simulink model "PubIfDecisionLM_MDL"  (R2020b)
settings: configuration reference "DspaceConfig" (kept outside this file)
PostLoadFcn:
  | if any(exist('dsrtsu_mdlpostloadfcn', 'file') ~= 0), dsrtsu_mdlpostloadfcn('Execute', bdroot); end
InitFcn:
  | , if any(exist('dsmpb_private', 'file') ~= 0), dsmpb_private('dsmpb_mdlclblib', 'Init', bdroot); end,
undefined symbols (not defined in the file or in its folder): OFM_OBJ_FUSIONTYPE_E, OFM_OBJ_MOVINGSTATE_E, OFM_OBJ_ORIENTATION_E, OFM_OBJ_TYPE_E, P_LM_Cyc, P_LM_EMLHistKapRcdBufSize, P_LM_EMLHistTrajBaseDis, P_LM_EMLHistTrajPNum, P_LM_EMLKapCorrMaxThre, P_LM_EMLMinKapThre, P_LM_EMLPathDisDiffThre, P_LM_EMLQuaFiltPar, P_LM_EMLTurnActKapThre, P_LM_EMLValidQuaThre, P_LM_FntPath1Disgap, P_LM_FntPath1MinDis, P_LM_FntPath1Timegap, P_LM_FntPath2Disgap, P_LM_FntPath2MinDis, P_LM_FntPath2Timegap, P_LM_FntPath3Disgap, P_LM_FntPath3MinDis, P_LM_FntPath3Timegap, P_LM_FusBLParFiltP, P_LM_FusEVDifC2Thre, P_LM_FusEVOPath1AllVSLDisThre, P_LM_FusEVOPath1AllVSLLostNumThre, P_LM_FusEVOPath1AllVSLQuaThre, P_LM_FusEVOPath1OTLFacNLC, P_LM_FusOTLQuaThre, P_LM_FusOTLSW, P_LM_FusParC0Index, P_LM_FusParC1Index, P_LM_FusParC2Index, P_LM_FusParC3Index, P_LM_FusVSLQuaThre, P_LM_FusVSLSW, P_LM_FusVSLValidSteerWheerAngThre, P_LM_FusVSLValidVxvThre, P_LM_LaneWidth, P_LM_OTLBufTPInfoEvaFactor, P_LM_OTLObjNum, P_LM_OTLObjSelectAgeThre, P_LM_OTLObjSelectDxAssessVx, P_LM_OTLObjSelectDxThre, P_LM_OTLObjSelectVxThre, P_LM_OTLObjSelectVyAssessDx, P_LM_OTLObjSelectVyThre, P_LM_OTLTrajPntBaseDis, P_LM_OTLTrajStdThre, P_LM_VSLAvailLineNum, P_LM_VSLBLSDiffThre, P_LM_VSLBLSDisRatio, P_LM_VSLFusBLParFiltP_C1, P_LM_VSLFusBLParFiltP_C2, P_LM_VSLFusBLParFiltP_C3, P_LM_VSLFusBLParFiltP_Quality, P_LM_VSLHistTrajBaseDis, P_LM_VSLHistTrajPNum, P_LM_VSLLCC0diff ... (+18)
libraries: simulink x145, LM_LIB x43
(part 13 of 24)

== system PubIfDecisionLM_MDL/Subsystem2/LM_OTL/LM_OTL_MovObjTrajRecord3/LM_OTL_MovObjSelc/LM_OTL_MovObjInterestedSelc/LM_OTL_ObjSelcIndexCalc ==
  ObjSelcDxInfo : Inport
  ObjSelcDyInfo : Inport  Port=2
  C_LM_ObjNum : Inport  Port=3
  LM_OTL_ObjSelcCalc : Subsystem
  LM_OTL_ObjSelcInfoOpt : Subsystem
  LeObj1CheckInfo : Outport
  LeObj2CheckInfo : Outport  Port=2
  HostObj1CheckInfo : Outport  Port=3
  HostObj2CheckInfo : Outport  Port=4
  RigObj1CheckInfo : Outport  Port=5
  RigObj2CheckInfo : Outport  Port=6
  wires:
  LM_OTL_ObjSelcCalc/4(HostObj2CheckInfo) -> HostObj2CheckInfo/1
  LM_OTL_ObjSelcCalc/1(LeObj1CheckInfo) -> LeObj1CheckInfo/1
  C_LM_ObjNum/1 -> LM_OTL_ObjSelcCalc/4(C_LM_ObjNum)
  ObjSelcDxInfo/1 -> LM_OTL_ObjSelcInfoOpt/1(ObjSelcDxInfo)
  LM_OTL_ObjSelcCalc/2(LeObj2CheckInfo) -> LeObj2CheckInfo/1
  ObjSelcDyInfo/1 -> LM_OTL_ObjSelcInfoOpt/2(ObjSelcDyInfo)
  LM_OTL_ObjSelcInfoOpt/3(RigObjSlecDxInfo) -> LM_OTL_ObjSelcCalc/3(RigObjSlecDxInfo)
  LM_OTL_ObjSelcInfoOpt/1(LeObjSelcDxInfo) -> LM_OTL_ObjSelcCalc/1(LeObjSelcDxInfo)
  LM_OTL_ObjSelcCalc/6(RigObj2CheckInfo) -> RigObj2CheckInfo/1
  LM_OTL_ObjSelcInfoOpt/2(HostObjSlecDxInfo) -> LM_OTL_ObjSelcCalc/2(HostObjSlecDxInfo)
  LM_OTL_ObjSelcCalc/5(RigObj1CheckInfo) -> RigObj1CheckInfo/1
  LM_OTL_ObjSelcCalc/3(HostObj1CheckInfo) -> HostObj1CheckInfo/1

== system PubIfDecisionLM_MDL/Subsystem2/LM_OTL/LM_OTL_MovObjTrajRecord3/LM_OTL_MovObjSelc/LM_OTL_MovObjInterestedSelc/LM_OTL_ObjSelcIndexCheck ==
  LeObj1CheckInfo : Inport
  LeObj2CheckInfo : Inport  Port=2
  HostObj1CheckInfo : Inport  Port=3
  HostObj2CheckInfo : Inport  Port=4
  RigObj1CheckInfo : Inport  Port=5
  RigObj2CheckInfo : Inport  Port=6
  LM_OTL_MovObjValid : Inport  Port=7
  Object_DX : Inport  Port=8
  HostObj1Check : Subsystem
  HostObj2Check : Subsystem
  LeObj1Check : Subsystem
  LeObj2Check : Subsystem
  RigObj1Check : Subsystem
  RigObj2Check : Subsystem
  LM_OTLLeObj1Index : Outport  PortDimensions=1
  LM_OTLLeObj2Index : Outport  Port=2  PortDimensions=1
  LM_OTLHostObj1Index : Outport  Port=3  PortDimensions=1
  LM_OTLHostObj2Index : Outport  Port=4  PortDimensions=1
  LM_OTLRigObj1Index : Outport  Port=5  PortDimensions=1
  LM_OTLRigObj2Index : Outport  Port=6  PortDimensions=1
  wires:
  LM_OTL_MovObjValid/1 -> RigObj2Check/1(LM_OTL_MovObjValid), RigObj1Check/1(LM_OTL_MovObjValid), HostObj2Check/1(LM_OTL_MovObjValid), HostObj1Check/1(LM_OTL_MovObjValid), LeObj2Check/1(LM_OTL_MovObjValid), LeObj1Check/1(LM_OTL_MovObjValid)
  Object_DX/1 -> LeObj1Check/2(Object_DX), LeObj2Check/2(Object_DX), HostObj1Check/2(Object_DX), HostObj2Check/2(Object_DX), RigObj1Check/2(Object_DX), RigObj2Check/2(Object_DX)
  RigObj2CheckInfo/1 -> RigObj2Check/3(RigObj2CheckInfo)
  RigObj2Check/1(LM_OTLRigObj2Index) -> LM_OTLRigObj2Index/1
  RigObj1CheckInfo/1 -> RigObj1Check/3(RigObj1CheckInfo)
  RigObj1Check/1(LM_OTLRigObj1Index) -> LM_OTLRigObj1Index/1
  HostObj2CheckInfo/1 -> HostObj2Check/3(HostObj2CheckInfo)
  HostObj2Check/1(LM_OTLHostObj2Index) -> LM_OTLHostObj2Index/1
  HostObj1CheckInfo/1 -> HostObj1Check/3(HostObj1CheckInfo)
  HostObj1Check/1(LM_OTLHostObj1Index) -> LM_OTLHostObj1Index/1
  LeObj2CheckInfo/1 -> LeObj2Check/3(LeObj2CheckInfo)
  LeObj2Check/1(LM_OTLLeObj2Index) -> LM_OTLLeObj2Index/1
  LeObj1Check/1(LM_OTLLeObj1Index) -> LM_OTLLeObj1Index/1
  LeObj1CheckInfo/1 -> LeObj1Check/3(LeObj1CheckInfo)

== system PubIfDecisionLM_MDL/Subsystem2/LM_OTL/LM_OTL_MovObjTrajRecord3/LM_OTL_MovObjSelc/LM_OTL_MovObjInterestedSelc/LM_OTL_ObjSelcInfoCalc ==
  ILM_OTL_MovObjValid : Inport
  Object_DX : Inport  Port=2
  Object_DY : Inport  Port=3
  C_LM_ObjNum : Inport  Port=4
  Constant1 : Constant  Value=255  OutDataTypeStr=single
  Constant2 : Constant  Value=255  OutDataTypeStr=single
  Index Vector : MultiPortSwitch  Inputs=1
  Index Vector1 : MultiPortSwitch  Inputs=1
  Index Vector2 : MultiPortSwitch  Inputs=1
  Switch6 : Switch  Criteria=u2 > Threshold
  Switch7 : Switch  Criteria=u2 > Threshold
  ObjSelcDxInfo : Outport
  ObjSelcDyInfo : Outport  Port=2
  wires:
  ILM_OTL_MovObjValid/1 -> Index Vector/2
  Object_DY/1 -> Index Vector2/2
  Switch6/1 -> ObjSelcDxInfo/1
  Constant2/1 -> Switch7/3
  Index Vector/1 -> Switch6/2, Switch7/2
  C_LM_ObjNum/1 -> Index Vector/1, Index Vector1/1, Index Vector2/1
  Index Vector1/1 -> Switch6/1
  Object_DX/1 -> Index Vector1/2
  Constant1/1 -> Switch6/3
  Switch7/1 -> ObjSelcDyInfo/1
  Index Vector2/1 -> Switch7/1

== system PubIfDecisionLM_MDL/Subsystem2/LM_OTL/LM_OTL_MovObjTrajRecord3/LM_OTL_MovObjSelc/Subsystem3/ILM_OTL_MovObjSelectDeFault ==
  Action Port : ActionPort  ActionPortLabel=if(u1)
  Constant : Constant  Value=0  OutDataTypeStr=boolean
  LM_OTL_MovObjValid : Outport
  wires:
  Constant/1 -> LM_OTL_MovObjValid/1

== system PubIfDecisionLM_MDL/Subsystem2/LM_OTL/LM_OTL_MovObjTrajRecord3/LM_OTL_MovObjSelc/Subsystem3/LM_OTL_MovObjSelect ==
  vxvRefMs : Inport
  Object_Type : Inport  Port=2
  Object_MovingState : Inport  Port=3
  Object_VX : Inport  Port=4
  Object_Orientation : Inport  Port=5
  Object_Fus_Type : Inport  Port=6
  Object_ExistProb : Inport  Port=7
  Object_VY : Inport  Port=8
  Object_DX : Inport  Port=9
  Object_Age : Inport  Port=10
  Action Port : ActionPort  ActionPortLabel=else
  LM_OTL_ExistProbAssess : Subsystem
  LM_OTL_FusTypeAssess : Subsystem
  LM_OTL_MovDirAssess : Subsystem
  LM_OTL_MovStsAssess : Subsystem
  LM_OTL_ObjAgeAssess : Subsystem
  LM_OTL_ObjDxAssess : Subsystem
  LM_OTL_ObjTypeAssess : Subsystem
  LM_OTL_ObjVyAssess : Subsystem
  Logical Operator : Logic  Inputs=8  AllPortsSameDT=off  OutDataTypeStr=boolean
  LM_OTL_MovObjValid : Outport
  wires:
  LM_OTL_ObjTypeAssess/1(LM_OTL_ObjTypeAssess) -> Logical Operator/1
  Object_Type/1 -> LM_OTL_ObjTypeAssess/1(Object_Type)
  LM_OTL_ObjDxAssess/1(LM_OTL_ObjDxValid) -> Logical Operator/7
  LM_OTL_ObjAgeAssess/1(LM_OTL_ObjAgeValid) -> Logical Operator/8
  LM_OTL_ObjVyAssess/1(LM_OTL_ObjVyValid) -> Logical Operator/6
  LM_OTL_ExistProbAssess/1(LM_OTL_ExistProbValid) -> Logical Operator/5
  LM_OTL_FusTypeAssess/1(LM_OTL_FusTypeValid) -> Logical Operator/4
  LM_OTL_MovDirAssess/1(LM_OTL_MovDirValid) -> Logical Operator/3
  LM_OTL_MovStsAssess/1(LM_OTL_MovStsValid) -> Logical Operator/2
  Object_VX/1 -> LM_OTL_MovStsAssess/2(Object_VX)
  Object_DX/1 -> LM_OTL_ObjVyAssess/2(Object_DX), LM_OTL_ObjDxAssess/1(Object_DX)
  Object_Orientation/1 -> LM_OTL_MovDirAssess/1(Object_Orientation)
  Object_MovingState/1 -> LM_OTL_MovStsAssess/1(Object_MovingState)
  Object_Age/1 -> LM_OTL_ObjAgeAssess/1(Object_Age)
  Object_Fus_Type/1 -> LM_OTL_FusTypeAssess/1(Object_Fus_Type), LM_OTL_ExistProbAssess/1(Object_Fus_Type)
  Logical Operator/1 -> LM_OTL_MovObjValid/1
  Object_ExistProb/1 -> LM_OTL_ExistProbAssess/2(Object_ExistProb)
  Object_VY/1 -> LM_OTL_ObjVyAssess/1(Object_VY)
  vxvRefMs/1 -> LM_OTL_MovStsAssess/3(vxvRefMs), LM_OTL_ObjDxAssess/2(vxvRefMs)

== system PubIfDecisionLM_MDL/Subsystem2/LM_OTL/LM_OTL_MovObjTrajRecord3/LM_OTL_MovObjSelc/Subsystem3/ObjIsInvalidCalc ==
  ObjectID : Inport
  Compare To Constant : simulink/Logic and Bit Operations/Compare To Constant  relop===  const=0  OutDataTypeStr=boolean
  ObjIsInvalid : Outport
  wires:
  Compare To Constant/1 -> ObjIsInvalid/1
  ObjectID/1 -> Compare To Constant/1

== system PubIfDecisionLM_MDL/Subsystem2/LM_OTL/LM_OTL_MovObjTrajRecord3/LM_OTL_ObjAlreadyRcdedJudge/LM_OTL_CurObjIDCalc/LM_OTL_CurEgoLaObjID ==
  Object_ID : Inport  BusOutputAsStruct=on
  LM_OTLCurEgoLaObj1Index : Inport  Port=2
  LM_OTLCurEgoLaObj2Index : Inport  Port=3
  Compare To Zero : simulink/Logic and Bit Operations/Compare To Zero  relop===  OutDataTypeStr=boolean
  Compare To Zero1 : simulink/Logic and Bit Operations/Compare To Zero  relop===  OutDataTypeStr=boolean
  Constant : Constant  Value=0  OutDataTypeStr=uint8
  Constant1 : Constant  OutDataTypeStr=uint8
  Constant2 : Constant  Value=0  OutDataTypeStr=uint8
  Constant3 : Constant  OutDataTypeStr=uint8
  Index Vector2 : MultiPortSwitch  Inputs=1
  Index Vector3 : MultiPortSwitch  Inputs=1
  Switch{,1..3} (4 alike) : Switch  Criteria=u2 ~= 0
  LM_OTLCurEgoLaObj1ID : Outport
  LM_OTLCurEgoLaObj2ID : Outport  Port=2
  wires:
  Switch1/1 -> Index Vector2/1
  LM_OTLCurEgoLaObj1Index/1 -> Switch1/3, Compare To Zero/1
  Constant/1 -> Switch/1
  Index Vector3/1 -> Switch2/3  "LM_Ego2ObjID"
  Compare To Zero1/1 -> Switch2/2, Switch3/2
  Constant3/1 -> Switch3/1
  Index Vector2/1 -> Switch/3  "LM_Ego1ObjID"
  Object_ID/1 -> Index Vector3/2, Index Vector2/2
  Switch/1 -> LM_OTLCurEgoLaObj1ID/1  "LM_OTLCurEgoLaObj1ID"
  LM_OTLCurEgoLaObj2Index/1 -> Compare To Zero1/1, Switch3/3
  Switch2/1 -> LM_OTLCurEgoLaObj2ID/1  "LM_OTLCurEgoLaObj2ID"
  Compare To Zero/1 -> Switch1/2, Switch/2
  Constant2/1 -> Switch2/1
  Switch3/1 -> Index Vector3/1
  Constant1/1 -> Switch1/1

== system PubIfDecisionLM_MDL/Subsystem2/LM_OTL/LM_OTL_MovObjTrajRecord3/LM_OTL_ObjAlreadyRcdedJudge/LM_OTL_CurObjIDCalc/LM_OTL_CurLeLaObjID ==
  Object_ID : Inport  BusOutputAsStruct=on
  LM_OTLCurLeLaObj1Index : Inport  Port=2
  LM_OTLCurLeLaObj2Index : Inport  Port=3
  Compare To Zero : simulink/Logic and Bit Operations/Compare To Zero  relop===  OutDataTypeStr=boolean
  Compare To Zero1 : simulink/Logic and Bit Operations/Compare To Zero  relop===  OutDataTypeStr=boolean
  Constant : Constant  Value=0  OutDataTypeStr=uint8
  Constant1 : Constant  OutDataTypeStr=uint8
  Constant2 : Constant  Value=0  OutDataTypeStr=uint8
  Constant3 : Constant  OutDataTypeStr=uint8
  Index Vector2 : MultiPortSwitch  Inputs=1
  Index Vector3 : MultiPortSwitch  Inputs=1
  Switch{,1..3} (4 alike) : Switch  Criteria=u2 ~= 0
  LM_OTLCurLeLaObj1ID : Outport
  LM_OTLCurLeLaObj2ID : Outport  Port=2
  wires:
  Index Vector3/1 -> Switch2/3  "LM_Le2ObjID"
  Index Vector2/1 -> Switch/3  "LM_Le1ObjID"
  Object_ID/1 -> Index Vector3/2, Index Vector2/2
  LM_OTLCurLeLaObj1Index/1 -> Switch1/3, Compare To Zero/1
  Compare To Zero/1 -> Switch1/2, Switch/2
  Switch/1 -> LM_OTLCurLeLaObj1ID/1  "LM_OTLCurLeLaObj1ID"
  Constant/1 -> Switch/1
  Switch1/1 -> Index Vector2/1
  Constant1/1 -> Switch1/1
  Constant2/1 -> Switch2/1
  Switch2/1 -> LM_OTLCurLeLaObj2ID/1  "LM_OTLCurLeLaObj2ID"
  Constant3/1 -> Switch3/1
  Compare To Zero1/1 -> Switch2/2, Switch3/2
  LM_OTLCurLeLaObj2Index/1 -> Compare To Zero1/1, Switch3/3
  Switch3/1 -> Index Vector3/1

== system PubIfDecisionLM_MDL/Subsystem2/LM_OTL/LM_OTL_MovObjTrajRecord3/LM_OTL_ObjAlreadyRcdedJudge/LM_OTL_CurObjIDCalc/LM_OTL_RigEgoLaObjID ==
  Object_ID : Inport  BusOutputAsStruct=on
  LM_OTLCurRigLaObj1Index : Inport  Port=2
  LM_OTLCurRigLaObj2Index : Inport  Port=3
  Compare To Zero : simulink/Logic and Bit Operations/Compare To Zero  relop===  OutDataTypeStr=boolean
  Compare To Zero1 : simulink/Logic and Bit Operations/Compare To Zero  relop===  OutDataTypeStr=boolean
  Constant : Constant  Value=0  OutDataTypeStr=uint8
  Constant1 : Constant  OutDataTypeStr=uint8
  Constant2 : Constant  Value=0  OutDataTypeStr=uint8
  Constant3 : Constant  OutDataTypeStr=uint8
  Index Vector2 : MultiPortSwitch  Inputs=1
  Index Vector3 : MultiPortSwitch  Inputs=1
  Switch{,1..3} (4 alike) : Switch  Criteria=u2 ~= 0
  LM_OTLCurRigLaObj1ID : Outport
  LM_OTLCurRigLaObj2ID : Outport  Port=2
  wires:
  Constant/1 -> Switch/1
  Compare To Zero1/1 -> Switch2/2, Switch3/2
  Index Vector3/1 -> Switch2/3  "LM_Rig2ObjID"
  Switch1/1 -> Index Vector2/1
  LM_OTLCurRigLaObj1Index/1 -> Switch1/3, Compare To Zero/1
  Constant1/1 -> Switch1/1
  Compare To Zero/1 -> Switch1/2, Switch/2
  Switch3/1 -> Index Vector3/1
  Constant2/1 -> Switch2/1
  Object_ID/1 -> Index Vector3/2, Index Vector2/2
  Switch/1 -> LM_OTLCurRigLaObj1ID/1  "LM_OTLCurRigLaObj1ID"
  Constant3/1 -> Switch3/1
  Index Vector2/1 -> Switch/3  "LM_Rig1ObjID"
  LM_OTLCurRigLaObj2Index/1 -> Compare To Zero1/1, Switch3/3
  Switch2/1 -> LM_OTLCurRigLaObj2ID/1  "LM_OTLCurRigLaObj2ID"

== system PubIfDecisionLM_MDL/Subsystem2/LM_OTL/LM_OTL_MovObjTrajRecord3/LM_OTL_ObjRcdFlgJudge/LM_OTL_CurObjDxCalc/LM_OTLCurEgoLaObjDxCalc ==
  LM_OTLCurEgoLaObj1Index : Inport
  Object_Dx : Inport  Port=2
  Object_Dy : Inport  Port=3
  LM_OTLCurEgoLaObj2Index : Inport  Port=4
  Compare To Zero : simulink/Logic and Bit Operations/Compare To Zero  relop===  OutDataTypeStr=boolean
  Compare To Zero1 : simulink/Logic and Bit Operations/Compare To Zero  relop===  OutDataTypeStr=boolean
  Constant : Constant  Value=0  OutDataTypeStr=single
  Constant8 : Constant  OutDataTypeStr=uint8
  Constant9 : Constant  OutDataTypeStr=uint8
  Index Vector{1..4} (4 alike) : MultiPortSwitch  Inputs=1
  Switch{1..6} (6 alike) : Switch  Criteria=u2 ~= 0
  LM_OTLCurEgoLaObj1Dx : Outport
  LM_OTLCurEgoLaObj1Dy : Outport  Port=2
  LM_OTLCurEgoLaObj2Dx : Outport  Port=3
  LM_OTLCurEgoLaObj2Dy : Outport  Port=4
  wires:
  Index Vector4/1 -> Switch4/3
  Switch4/1 -> LM_OTLCurEgoLaObj2Dy/1  "LM_OTLCurEgoLaObj2Dy"
  Index Vector1/1 -> Switch3/3
  Object_Dy/1 -> Index Vector1/2, Index Vector4/2
  Switch3/1 -> LM_OTLCurEgoLaObj1Dy/1  "LM_OTLCurEgoLaObj1Dy"
  Index Vector3/1 -> Switch2/3
  Constant/1 -> Switch1/1, Switch2/1, Switch4/1, Switch3/1
  Switch1/1 -> LM_OTLCurEgoLaObj1Dx/1  "LM_OTLCurEgoLaObj1Dx"
  Switch2/1 -> LM_OTLCurEgoLaObj2Dx/1  "LM_OTLCurEgoLaObj2Dx"
  Index Vector2/1 -> Switch1/3
  Switch5/1 -> Index Vector2/1, Index Vector1/1
  Switch6/1 -> Index Vector3/1, Index Vector4/1
  Constant9/1 -> Switch6/1
  Compare To Zero/1 -> Switch5/2, Switch1/2, Switch3/2
  Compare To Zero1/1 -> Switch6/2, Switch2/2, Switch4/2
  Constant8/1 -> Switch5/1
  Object_Dx/1 -> Index Vector3/2, Index Vector2/2
  LM_OTLCurEgoLaObj1Index/1 -> Compare To Zero/1, Switch5/3
  LM_OTLCurEgoLaObj2Index/1 -> Switch6/3, Compare To Zero1/1

== system PubIfDecisionLM_MDL/Subsystem2/LM_OTL/LM_OTL_MovObjTrajRecord3/LM_OTL_ObjRcdFlgJudge/LM_OTL_CurObjDxCalc/LM_OTLCurLeLaObjDxCalc ==
  LM_OTLCurLeLaObj1Index : Inport
  Object_Dx : Inport  Port=2
  Object_Dy : Inport  Port=3
  LM_OTLCurLeLaObj2Index : Inport  Port=4
  Compare To Zero : simulink/Logic and Bit Operations/Compare To Zero  relop===  OutDataTypeStr=boolean
  Compare To Zero1 : simulink/Logic and Bit Operations/Compare To Zero  relop===  OutDataTypeStr=boolean
  Constant : Constant  Value=0  OutDataTypeStr=single
  Constant8 : Constant  OutDataTypeStr=uint8
  Constant9 : Constant  OutDataTypeStr=uint8
  Index Vector{1..4} (4 alike) : MultiPortSwitch  Inputs=1
  Switch{1..6} (6 alike) : Switch  Criteria=u2 ~= 0
  LM_OTLCurLeLaObj1Dx : Outport
  LM_OTLCurLeLaObj1Dy : Outport  Port=2
  LM_OTLCurLeLaObj2Dx : Outport  Port=3
  LM_OTLCurLeLaObj2Dy : Outport  Port=4
  wires:
  LM_OTLCurLeLaObj2Index/1 -> Compare To Zero1/1, Switch6/3
  LM_OTLCurLeLaObj1Index/1 -> Switch5/3, Compare To Zero/1
  Object_Dx/1 -> Index Vector2/2, Index Vector3/2
  Constant8/1 -> Switch5/1
  Compare To Zero1/1 -> Switch4/2, Switch2/2, Switch6/2
  Compare To Zero/1 -> Switch3/2, Switch1/2, Switch5/2
  Constant9/1 -> Switch6/1
  Switch6/1 -> Index Vector4/1, Index Vector3/1
  Switch5/1 -> Index Vector1/1, Index Vector2/1
  Index Vector2/1 -> Switch1/3
  Switch2/1 -> LM_OTLCurLeLaObj2Dx/1  "LM_OTLCurLeLaObj2Dx"
  Switch1/1 -> LM_OTLCurLeLaObj1Dx/1  "LM_OTLCurLeLaObj1Dx"
  Constant/1 -> Switch3/1, Switch4/1, Switch2/1, Switch1/1
  Index Vector3/1 -> Switch2/3
  Switch3/1 -> LM_OTLCurLeLaObj1Dy/1  "LM_OTLCurLeLaObj1Dy"
  Object_Dy/1 -> Index Vector4/2, Index Vector1/2
  Index Vector1/1 -> Switch3/3
  Switch4/1 -> LM_OTLCurLeLaObj2Dy/1  "LM_OTLCurLeLaObj2Dy"
  Index Vector4/1 -> Switch4/3

== system PubIfDecisionLM_MDL/Subsystem2/LM_OTL/LM_OTL_MovObjTrajRecord3/LM_OTL_ObjRcdFlgJudge/LM_OTL_CurObjDxCalc/LM_OTLCurRigLaObjDxCalc ==
  LM_OTLCurRigLaObj1Index : Inport
  Object_Dx : Inport  Port=2
  Object_Dy : Inport  Port=3
  LM_OTLCurRigLaObj2Index : Inport  Port=4
  Compare To Zero : simulink/Logic and Bit Operations/Compare To Zero  relop===  OutDataTypeStr=boolean
  Compare To Zero1 : simulink/Logic and Bit Operations/Compare To Zero  relop===  OutDataTypeStr=boolean
  Constant : Constant  Value=0  OutDataTypeStr=single
  Constant8 : Constant  OutDataTypeStr=uint8
  Constant9 : Constant  OutDataTypeStr=uint8
  Index Vector{1..4} (4 alike) : MultiPortSwitch  Inputs=1
  Switch{1..6} (6 alike) : Switch  Criteria=u2 ~= 0
  LM_OTLCurRigLaObj1Dx : Outport
  LM_OTLCurRigLaObj1Dy : Outport  Port=2
  LM_OTLCurRigLaObj2Dx : Outport  Port=3
  LM_OTLCurRigLaObj2Dy : Outport  Port=4
  wires:
  LM_OTLCurRigLaObj2Index/1 -> Compare To Zero1/1, Switch6/3
  LM_OTLCurRigLaObj1Index/1 -> Switch5/3, Compare To Zero/1
  Object_Dx/1 -> Index Vector2/2, Index Vector3/2
  Constant8/1 -> Switch5/1
  Compare To Zero1/1 -> Switch4/2, Switch2/2, Switch6/2
  Compare To Zero/1 -> Switch3/2, Switch1/2, Switch5/2
  Constant9/1 -> Switch6/1
  Switch6/1 -> Index Vector4/1, Index Vector3/1
  Switch5/1 -> Index Vector1/1, Index Vector2/1
  Index Vector2/1 -> Switch1/3
  Switch2/1 -> LM_OTLCurRigLaObj2Dx/1  "LM_OTLCurRigLaObj2Dx"
  Switch1/1 -> LM_OTLCurRigLaObj1Dx/1  "LM_OTLCurRigLaObj1Dx"
  Constant/1 -> Switch3/1, Switch4/1, Switch2/1, Switch1/1
  Index Vector3/1 -> Switch2/3
  Switch3/1 -> LM_OTLCurRigLaObj1Dy/1  "LM_OTLCurRigLaObj1Dy"
  Object_Dy/1 -> Index Vector4/2, Index Vector1/2
  Index Vector1/1 -> Switch3/3
  Switch4/1 -> LM_OTLCurRigLaObj2Dy/1  "LM_OTLCurRigLaObj2Dy"
  Index Vector4/1 -> Switch4/3

== system PubIfDecisionLM_MDL/Subsystem2/LM_OTL/LM_OTL_MovObjTrajRecord3/LM_OTL_ObjStoreInfoCalc/LM_OTL_BufLe1InfoUpdate1/LM_OTL_BufLe1InfoUpdate ==
  LM_OTLBufL1DxVectK1Adju : Inport
  LM_OTLBufL1DyVectK1Adju : Inport  Port=2
  LM_OTLBufL1UpdateFlg : Inport  Port=3
  LM_OTLBufL1Objdx : Inport  Port=4
  LM_OTLBufL1Objdy : Inport  Port=5
  LM_OTLBufL1EPPos : Inport  Port=6
  If : If  IfExpression=u1 ~= 0
  If Action Subsystem : Subsystem  TreatAsAtomicUnit=on
  If Action Subsystem1 : Subsystem  TreatAsAtomicUnit=on
  Merge : Merge
  Merge1 : Merge
  LM_OTLBufL1DxVect : Outport  PortDimensions=80
  LM_OTLBufL1DyVect : Outport  Port=2  PortDimensions=80
  wires:
  Merge1/1 -> LM_OTLBufL1DyVect/1  "LM_OTLBufL1DyVect"
  If Action Subsystem1/2(LM_OTLBufL1DyVect) -> Merge1/2
  If Action Subsystem/2(LM_OTLBufL1DyVect) -> Merge1/1
  Merge/1 -> LM_OTLBufL1DxVect/1  "LM_OTLBufL1DxVect"
  If Action Subsystem1/1(LM_OTLBufL1DxVect) -> Merge/2
  If Action Subsystem/1(LM_OTLBufL1DxVect) -> Merge/1
  LM_OTLBufL1EPPos/1 -> If Action Subsystem/3(LM_OTLBufL1EPPos)
  LM_OTLBufL1Objdy/1 -> If Action Subsystem/2(LM_OTLBufL1Objdy)
  LM_OTLBufL1Objdx/1 -> If Action Subsystem/1(LM_OTLBufL1Objdx)
  LM_OTLBufL1DyVectK1Adju/1 -> If Action Subsystem1/2(LM_OTLBufL1DyVectK1Adju), If Action Subsystem/5(LM_OTLBufL1DyVectK1Adju)
  LM_OTLBufL1DxVectK1Adju/1 -> If Action Subsystem1/1(LM_OTLBufL1DxVectK1Adju), If Action Subsystem/4(LM_OTLBufL1DxVectK1Adju)
  If/2 -> If Action Subsystem1/Action
  If/1 -> If Action Subsystem/Action
  LM_OTLBufL1UpdateFlg/1 -> If/1

== system PubIfDecisionLM_MDL/Subsystem2/LM_OTL/LM_OTL_MovObjTrajRecord3/LM_OTL_ObjStoreInfoCalc/LM_OTL_BufLe1InfoUpdate1/LM_OTL_BufLe1StoreInfoCalc ==
  LM_OTLBufIndex : Inport
  LM_OTLCurLeLaObj1RcdedFlg : Inport  Port=2
  LM_OTLCurLeLaObj2RcdedFlg : Inport  Port=3
  LM_OTLCurLeLaObj1RcdFlg : Inport  Port=4
  LM_OTLCurLeLaObj2RcdFlg : Inport  Port=5
  LM_OTLCurLeLaObj1ID : Inport  Port=6
  LM_OTLCurLeLaObj2ID : Inport  Port=7
  LM_OTLCurLeLaObj1Dx : Inport  Port=8
  LM_OTLCurLeLaObj2Dx : Inport  Port=9
  LM_OTLCurLeLaObj1Dy : Inport  Port=10
  LM_OTLCurLeLaObj2Dy : Inport  Port=11
  LM_OTLBufL1PNumK1 : Inport  Port=12
  LM_OTLBufL1SPPosK1 : Inport  Port=13
  LM_OTLBufL1EPPosK1 : Inport  Port=14
  LM_OTLCurLeLaObj1Index : Inport  Port=15
  LM_OTLCurLeLaObj2Index : Inport  Port=16
  LM_OTLBufL1LastTPValid : Inport  Port=17
  LM_OTLBufL1LastEPPos : Inport  Port=18
  If : If  NumInputs=3  IfExpression=u1 == u2  ElseIfExpressions=u2 == u3
  LM_OTL_ObjSICCurLeObj1InBufLe1 : Subsystem
  LM_OTL_ObjSICCurLeObj2InBufLe1 : Subsystem
  LM_OTL_ObjSICNoCurObjInBufLe1 : Subsystem
  Merge{,1..6} (7 alike) : Merge  Inputs=3
  LM_OTLBufL1UpdateFlg : Outport
  LM_OTLBufL1Objdx : Outport  Port=2
  LM_OTLBufL1Objdy : Outport  Port=3
  LM_OTLBufL1EPPos : Outport  Port=4
  LM_OTLBufL1ObjID : Outport  Port=5
  LM_OTLBufL1ObjTPNum : Outport  Port=6
  LM_OTLBufL1SPPos : Outport  Port=7
  wires:
  LM_OTLBufIndex/1 -> If/1
  If/1 -> LM_OTL_ObjSICCurLeObj1InBufLe1/Action
  If/2 -> LM_OTL_ObjSICCurLeObj2InBufLe1/Action
  If/3 -> LM_OTL_ObjSICNoCurObjInBufLe1/Action
  LM_OTLCurLeLaObj1RcdedFlg/1 -> LM_OTL_ObjSICNoCurObjInBufLe1/3(LM_OTLCurLeLaObj1RcdedFlg), If/2
  LM_OTLCurLeLaObj2RcdedFlg/1 -> If/3
  LM_OTLCurLeLaObj1RcdFlg/1 -> LM_OTL_ObjSICCurLeObj1InBufLe1/1(LM_OTLCurLeLaObj1RcdFlg)
  LM_OTLCurLeLaObj1ID/1 -> LM_OTL_ObjSICNoCurObjInBufLe1/4(LM_OTLCurLeLaObj1ID), LM_OTL_ObjSICCurLeObj1InBufLe1/2(LM_OTLCurLeLaObj1ID)
  LM_OTLCurLeLaObj1Dx/1 -> LM_OTL_ObjSICNoCurObjInBufLe1/6(LM_OTLCurLeLaObj1Dx), LM_OTL_ObjSICCurLeObj1InBufLe1/3(LM_OTLCurLeLaObj1Dx)
  LM_OTLCurLeLaObj1Dy/1 -> LM_OTL_ObjSICNoCurObjInBufLe1/8(LM_OTLCurLeLaObj1Dy), LM_OTL_ObjSICCurLeObj1InBufLe1/4(LM_OTLCurLeLaObj1Dy)
  LM_OTLBufL1PNumK1/1 -> LM_OTL_ObjSICCurLeObj2InBufLe1/5(LM_OTLBufL1PNumK1), LM_OTL_ObjSICCurLeObj1InBufLe1/5(LM_OTLBufL1PNumK1)
  LM_OTLBufL1SPPosK1/1 -> LM_OTL_ObjSICCurLeObj2InBufLe1/6(LM_OTLBufL1SPPosK1), LM_OTL_ObjSICCurLeObj1InBufLe1/6(LM_OTLBufL1SPPosK1)
  LM_OTLBufL1EPPosK1/1 -> LM_OTL_ObjSICCurLeObj2InBufLe1/7(LM_OTLBufL1EPPosK1), LM_OTL_ObjSICCurLeObj1InBufLe1/7(LM_OTLBufL1EPPosK1)
  LM_OTLCurLeLaObj2RcdFlg/1 -> LM_OTL_ObjSICCurLeObj2InBufLe1/1(LM_OTLCurLeLaObj2RcdFlg)
  LM_OTLCurLeLaObj2ID/1 -> LM_OTL_ObjSICCurLeObj2InBufLe1/2(LM_OTLCurLeLaObj2ID), LM_OTL_ObjSICNoCurObjInBufLe1/5(LM_OTLCurLeLaObj2ID)
  LM_OTLCurLeLaObj2Dx/1 -> LM_OTL_ObjSICNoCurObjInBufLe1/7(LM_OTLCurLeLaObj2Dx), LM_OTL_ObjSICCurLeObj2InBufLe1/3(LM_OTLCurLeLaObj2Dx)
  LM_OTLCurLeLaObj2Dy/1 -> LM_OTL_ObjSICNoCurObjInBufLe1/9(LM_OTLCurLeLaObj2Dy), LM_OTL_ObjSICCurLeObj2InBufLe1/4(LM_OTLCurLeLaObj2Dy)
  LM_OTL_ObjSICCurLeObj1InBufLe1/1(LM_OTLBufL1UpdateFlg) -> Merge/1
  Merge/1 -> LM_OTLBufL1UpdateFlg/1
  LM_OTL_ObjSICCurLeObj1InBufLe1/2(LM_OTLBufL1ObjID) -> Merge1/1
  Merge1/1 -> LM_OTLBufL1ObjID/1
  LM_OTL_ObjSICCurLeObj1InBufLe1/3(LM_OTLBufL1Objdx) -> Merge2/1
  Merge2/1 -> LM_OTLBufL1Objdx/1
  LM_OTL_ObjSICCurLeObj1InBufLe1/4(LM_OTLBufL1Objdy) -> Merge3/1
  Merge3/1 -> LM_OTLBufL1Objdy/1
  LM_OTL_ObjSICCurLeObj1InBufLe1/5(LM_OTLBufL1ObjTPNum) -> Merge4/1
  Merge4/1 -> LM_OTLBufL1ObjTPNum/1
  LM_OTL_ObjSICCurLeObj1InBufLe1/6(LM_OTLBufL1ObjTPSP) -> Merge5/1
  Merge5/1 -> LM_OTLBufL1SPPos/1
  LM_OTL_ObjSICCurLeObj1InBufLe1/7(LM_OTLBufL1ObjTPEP) -> Merge6/1
  Merge6/1 -> LM_OTLBufL1EPPos/1
  LM_OTL_ObjSICCurLeObj2InBufLe1/1(LM_OTLBufL1UpdateFlg) -> Merge/2
  LM_OTL_ObjSICCurLeObj2InBufLe1/2(LM_OTLBufL1ObjID) -> Merge1/2
  LM_OTL_ObjSICCurLeObj2InBufLe1/3(LM_OTLBufL1Objdx) -> Merge2/2
  LM_OTL_ObjSICCurLeObj2InBufLe1/4(LM_OTLBufL1Objdy) -> Merge3/2
  LM_OTL_ObjSICCurLeObj2InBufLe1/5(LM_OTLBufL1ObjTPNum) -> Merge4/2
  LM_OTL_ObjSICCurLeObj2InBufLe1/6(LM_OTLBufL1ObjTPSP) -> Merge5/2
  LM_OTL_ObjSICCurLeObj2InBufLe1/7(LM_OTLBufL1ObjTPEP) -> Merge6/2
  LM_OTL_ObjSICNoCurObjInBufLe1/1(LM_OTLBufL1UpdateFlg) -> Merge/3
  LM_OTL_ObjSICNoCurObjInBufLe1/2(LM_OTLBufL1ObjID) -> Merge1/3
  LM_OTL_ObjSICNoCurObjInBufLe1/3(LM_OTLBufL1Objdx) -> Merge2/3
  LM_OTL_ObjSICNoCurObjInBufLe1/4(LM_OTLBufL1Objdy) -> Merge3/3
  LM_OTL_ObjSICNoCurObjInBufLe1/5(LM_OTLBufL1ObjTPNum) -> Merge4/3
  LM_OTL_ObjSICNoCurObjInBufLe1/6(LM_OTLBufL1ObjTPSP) -> Merge5/3
  LM_OTL_ObjSICNoCurObjInBufLe1/7(LM_OTLBufL1ObjTPEP) -> Merge6/3
  LM_OTLCurLeLaObj1Index/1 -> LM_OTL_ObjSICNoCurObjInBufLe1/1(LM_OTLCurLeLaObj1Index)
  LM_OTLCurLeLaObj2Index/1 -> LM_OTL_ObjSICNoCurObjInBufLe1/2(LM_OTLCurLeLaObj2Index)
  LM_OTLBufL1LastTPValid/1 -> LM_OTL_ObjSICNoCurObjInBufLe1/10(LM_OTLBufL1LastTPValid)
  LM_OTLBufL1LastEPPos/1 -> LM_OTL_ObjSICNoCurObjInBufLe1/11(LM_OTLBufL1LastEPPos)

== system PubIfDecisionLM_MDL/Subsystem2/LM_OTL/LM_OTL_MovObjTrajRecord3/LM_OTL_ObjStoreInfoCalc/Subsystem/LM_OTL_BufEPPosInfo ==
  LM_OTLBufL1EPPos : Inport
  LM_OTLBufL2EPPos : Inport  Port=2
  LM_OTLBufE1EPPos : Inport  Port=3
  LM_OTLBufE2EPPos : Inport  Port=4
  LM_OTLBufR1EPPos : Inport  Port=5
  LM_OTLBufR2EPPos : Inport  Port=6
  Bus Creator5 : BusCreator  Inputs=6
  LM_OTLBufEPPosInfo : Outport
  wires:
  Bus Creator5/1 -> LM_OTLBufEPPosInfo/1  "LM_OTLBufEPPosInfo"
  LM_OTLBufL2EPPos/1 -> Bus Creator5/2  "LM_OTLBufL2EPPos"
  LM_OTLBufR2EPPos/1 -> Bus Creator5/6  "LM_OTLBufR2EPPos"
  LM_OTLBufR1EPPos/1 -> Bus Creator5/5  "LM_OTLBufR1EPPos"
  LM_OTLBufL1EPPos/1 -> Bus Creator5/1  "LM_OTLBufL1EPPos"
  LM_OTLBufE2EPPos/1 -> Bus Creator5/4  "LM_OTLBufE2EPPos"
  LM_OTLBufE1EPPos/1 -> Bus Creator5/3  "LM_OTLBufE1EPPos"

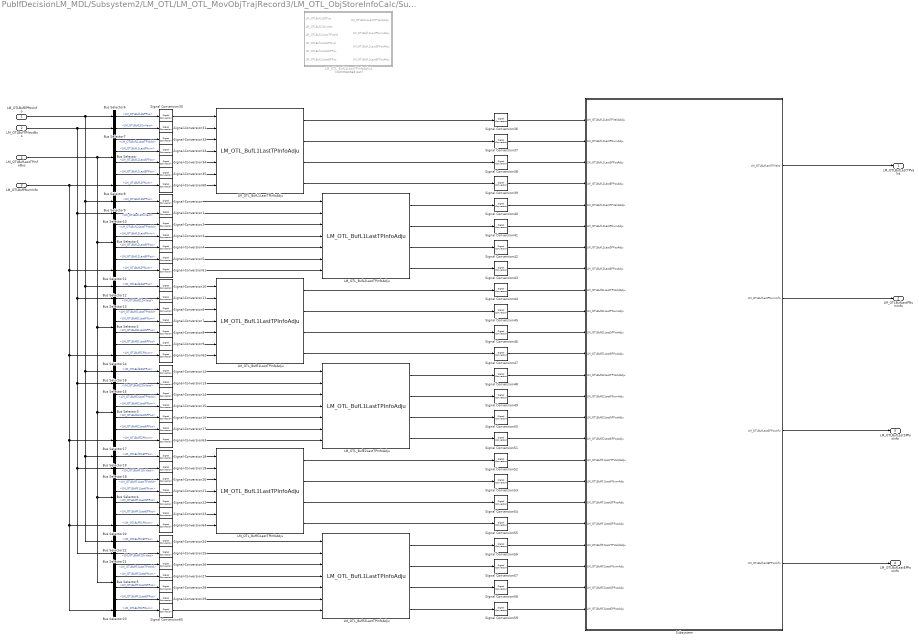
== system PubIfDecisionLM_MDL/Subsystem2/LM_OTL/LM_OTL_MovObjTrajRecord3/LM_OTL_ObjStoreInfoCalc/Subsystem/LM_OTL_BufLastTPInfo ==
  LM_OTLBufEPPosInfo : Inport
  LM_OTLBufTPVectBus : Inport  Port=2
  LM_OTLBufPNumInfo : Inport  Port=3
  LM_OTLBufLastTPInfoBus : Inport  Port=4
  Bus Selector : BusSelector  OutputSignals=LM_OTLBufL1LastTPInfo.LM_OTLBufL1LastTPValid,LM_OTLBufL1LastTPInfo.LM_OTLBufL1LastPNum,LM_OTLBufL1LastTPInfo.LM_OTLBufL1LastSPPos,LM_OTLBufL1LastTPInfo.LM_OTLBufL1LastEPPos
  Bus Selector1 : BusSelector  OutputSignals=LM_OTLBufL2LastTPInfo.LM_OTLBufL2LastTPValid,LM_OTLBufL2LastTPInfo.LM_OTLBufL2LastPNum,LM_OTLBufL2LastTPInfo.LM_OTLBufL2LastSPPos,LM_OTLBufL2LastTPInfo.LM_OTLBufL2LastEPPos
  Bus Selector10 : BusSelector  OutputSignals=LM_OTLBufL2DxVect
  Bus Selector11 : BusSelector  OutputSignals=LM_OTLBufL2PNum
  Bus Selector12 : BusSelector  OutputSignals=LM_OTLBufE1EPPos
  Bus Selector13 : BusSelector  OutputSignals=LM_OTLBufE1DxVect
  Bus Selector14 : BusSelector  OutputSignals=LM_OTLBufE1PNum
  Bus Selector15 : BusSelector  OutputSignals=LM_OTLBufE2DxVect
  Bus Selector16 : BusSelector  OutputSignals=LM_OTLBufE2EPPos
  Bus Selector17 : BusSelector  OutputSignals=LM_OTLBufE2PNum
  Bus Selector18 : BusSelector  OutputSignals=LM_OTLBufR1DxVect
  Bus Selector19 : BusSelector  OutputSignals=LM_OTLBufR1EPPos
  Bus Selector2 : BusSelector  OutputSignals=LM_OTLBufE1LastTPInfo.LM_OTLBufE1LastTPValid,LM_OTLBufE1LastTPInfo.LM_OTLBufE1LastPNum,LM_OTLBufE1LastTPInfo.LM_OTLBufE1LastSPPos,LM_OTLBufE1LastTPInfo.LM_OTLBufE1LastEPPos
  Bus Selector20 : BusSelector  OutputSignals=LM_OTLBufR1PNum
  Bus Selector21 : BusSelector  OutputSignals=LM_OTLBufR2DxVect
  Bus Selector22 : BusSelector  OutputSignals=LM_OTLBufR2EPPos
  Bus Selector23 : BusSelector  OutputSignals=LM_OTLBufR2PNum
  Bus Selector3 : BusSelector  OutputSignals=LM_OTLBufE2LastTPInfo.LM_OTLBufE2LastTPValid,LM_OTLBufE2LastTPInfo.LM_OTLBufE2LastPNum,LM_OTLBufE2LastTPInfo.LM_OTLBufE2LastSPPos,LM_OTLBufE2LastTPInfo.LM_OTLBufE2LastEPPos
  Bus Selector4 : BusSelector  OutputSignals=LM_OTLBufR1LastTPInfo.LM_OTLBufR1LastTPValid,LM_OTLBufR1LastTPInfo.LM_OTLBufR1LastPNum,LM_OTLBufR1LastTPInfo.LM_OTLBufR1LastSPPos,LM_OTLBufR1LastTPInfo.LM_OTLBufR1LastEPPos
  Bus Selector5 : BusSelector  OutputSignals=LM_OTLBufR2LastTPInfo.LM_OTLBufR2LastTPValid,LM_OTLBufR2LastTPInfo.LM_OTLBufR2LastPNum,LM_OTLBufR2LastTPInfo.LM_OTLBufR2LastSPPos,LM_OTLBufR2LastTPInfo.LM_OTLBufR2LastEPPos
  Bus Selector6 : BusSelector  OutputSignals=LM_OTLBufL1EPPos
  Bus Selector7 : BusSelector  OutputSignals=LM_OTLBufL1DxVect
  Bus Selector8 : BusSelector  OutputSignals=LM_OTLBufL1PNum
  Bus Selector9 : BusSelector  OutputSignals=LM_OTLBufL2EPPos
  LM_OTL_BufE1LastTPInfoAdju : LM_LIB/LM_OTL_BufL1LastTPInfoAdju  SystemSampleTime=-1  VariantActivationTime=update diagram  Latency=0  AutoFrameSizeCalculation=off
  LM_OTL_BufE2LastTPInfoAdju : LM_LIB/LM_OTL_BufL1LastTPInfoAdju  SystemSampleTime=-1  VariantActivationTime=update diagram  Latency=0  AutoFrameSizeCalculation=off
  LM_OTL_BufL1LastTPInfoAdju : LM_LIB/LM_OTL_BufL1LastTPInfoAdju  SystemSampleTime=-1  VariantActivationTime=update diagram  Latency=0  AutoFrameSizeCalculation=off
  LM_OTL_BufL1LastTPInfoAdju1 : Subsystem  Commented=on
  LM_OTL_BufL2LastTPInfoAdju : LM_LIB/LM_OTL_BufL1LastTPInfoAdju  SystemSampleTime=-1  VariantActivationTime=update diagram  Latency=0  AutoFrameSizeCalculation=off
  LM_OTL_BufR1LastTPInfoAdju : LM_LIB/LM_OTL_BufL1LastTPInfoAdju  SystemSampleTime=-1  VariantActivationTime=update diagram  Latency=0  AutoFrameSizeCalculation=off
  LM_OTL_BufR2LastTPInfoAdju : LM_LIB/LM_OTL_BufL1LastTPInfoAdju  SystemSampleTime=-1  VariantActivationTime=update diagram  Latency=0  AutoFrameSizeCalculation=off
  Signal Conversion{,1..65} (66 alike) : SignalConversion  OverrideOpt=off
  Subsystem : Subsystem
  LM_OTLBufLastTPValid : Outport
  LM_OTLBufLastPNumInfo : Outport  Port=2
  LM_OTLBufLastSPPosInfo : Outport  Port=3
  LM_OTLBufLastEPPosInfo : Outport  Port=4
  wires:
  Signal Conversion65/1 -> LM_OTL_BufR2LastTPInfoAdju/7
  Bus Selector23/1 -> Signal Conversion65/1  "<LM_OTLBufR2PNum>"
  Bus Selector21/1 -> Signal Conversion25/1  "<LM_OTLBufR2DxVect>"
  Bus Selector22/1 -> Signal Conversion24/1  "<LM_OTLBufR2EPPos>"
  LM_OTLBufTPVectBus/1 -> Bus Selector7/1, Bus Selector10/1, Bus Selector13/1, Bus Selector15/1, Bus Selector18/1, Bus Selector21/1
  LM_OTLBufEPPosInfo/1 -> Bus Selector6/1, Bus Selector9/1, Bus Selector12/1, Bus Selector16/1, Bus Selector19/1, Bus Selector22/1
  Signal Conversion64/1 -> LM_OTL_BufR1LastTPInfoAdju/7
  Bus Selector20/1 -> Signal Conversion64/1  "<LM_OTLBufR1PNum>"
  Bus Selector19/1 -> Signal Conversion18/1  "<LM_OTLBufR1EPPos>"
  Bus Selector18/1 -> Signal Conversion19/1  "<LM_OTLBufR1DxVect>"
  Signal Conversion63/1 -> LM_OTL_BufE2LastTPInfoAdju/7
  Bus Selector17/1 -> Signal Conversion63/1  "<LM_OTLBufE2PNum>"
  Bus Selector15/1 -> Signal Conversion13/1  "<LM_OTLBufE2DxVect>"
  Bus Selector16/1 -> Signal Conversion12/1  "<LM_OTLBufE2EPPos>"
  Signal Conversion62/1 -> LM_OTL_BufE1LastTPInfoAdju/7
  Bus Selector14/1 -> Signal Conversion62/1  "<LM_OTLBufE1PNum>"
  Signal Conversion61/1 -> LM_OTL_BufL2LastTPInfoAdju/7
  Bus Selector11/1 -> Signal Conversion61/1  "<LM_OTLBufL2PNum>"
  Bus Selector10/1 -> Signal Conversion1/1  "<LM_OTLBufL2DxVect>"
  Bus Selector9/1 -> Signal Conversion/1  "<LM_OTLBufL2EPPos>"
  LM_OTLBufPNumInfo/1 -> Bus Selector8/1, Bus Selector11/1, Bus Selector14/1, Bus Selector17/1, Bus Selector23/1, Bus Selector20/1
  Bus Selector8/1 -> Signal Conversion60/1  "<LM_OTLBufL1PNum>"
  Bus Selector7/1 -> Signal Conversion31/1  "<LM_OTLBufL1DxVect>"
  Bus Selector6/1 -> Signal Conversion30/1  "<LM_OTLBufL1EPPos>"
  Signal Conversion60/1 -> LM_OTL_BufL1LastTPInfoAdju/7
  Bus Selector/1 -> Signal Conversion32/1  "<LM_OTLBufL1LastTPValid>"
  Bus Selector/2 -> Signal Conversion33/1  "<LM_OTLBufL1LastPNum>"
  Bus Selector/3 -> Signal Conversion34/1  "<LM_OTLBufL1LastSPPos>"
  Bus Selector/4 -> Signal Conversion35/1  "<LM_OTLBufL1LastEPPos>"
  Signal Conversion/1 -> LM_OTL_BufL2LastTPInfoAdju/1
  Signal Conversion1/1 -> LM_OTL_BufL2LastTPInfoAdju/2
  Bus Selector1/2 -> Signal Conversion3/1  "<LM_OTLBufL2LastPNum>"
  Bus Selector1/1 -> Signal Conversion2/1  "<LM_OTLBufL2LastTPValid>"
  Bus Selector1/3 -> Signal Conversion4/1  "<LM_OTLBufL2LastSPPos>"
  Bus Selector1/4 -> Signal Conversion5/1  "<LM_OTLBufL2LastEPPos>"
  Bus Selector12/1 -> Signal Conversion10/1  "<LM_OTLBufE1EPPos>"
  Bus Selector13/1 -> Signal Conversion11/1  "<LM_OTLBufE1DxVect>"
  Signal Conversion2/1 -> LM_OTL_BufL2LastTPInfoAdju/3
  Signal Conversion3/1 -> LM_OTL_BufL2LastTPInfoAdju/4
  Signal Conversion4/1 -> LM_OTL_BufL2LastTPInfoAdju/5
  Signal Conversion5/1 -> LM_OTL_BufL2LastTPInfoAdju/6
  Signal Conversion9/1 -> LM_OTL_BufE1LastTPInfoAdju/6
  Signal Conversion8/1 -> LM_OTL_BufE1LastTPInfoAdju/5
  Signal Conversion7/1 -> LM_OTL_BufE1LastTPInfoAdju/4
  Signal Conversion6/1 -> LM_OTL_BufE1LastTPInfoAdju/3
  Bus Selector2/4 -> Signal Conversion9/1  "<LM_OTLBufE1LastEPPos>"
  Bus Selector2/3 -> Signal Conversion8/1  "<LM_OTLBufE1LastSPPos>"
  Bus Selector2/1 -> Signal Conversion6/1  "<LM_OTLBufE1LastTPValid>"
  Bus Selector2/2 -> Signal Conversion7/1  "<LM_OTLBufE1LastPNum>"
  Signal Conversion10/1 -> LM_OTL_BufE1LastTPInfoAdju/1
  Signal Conversion11/1 -> LM_OTL_BufE1LastTPInfoAdju/2
  Signal Conversion13/1 -> LM_OTL_BufE2LastTPInfoAdju/2
  Signal Conversion12/1 -> LM_OTL_BufE2LastTPInfoAdju/1
  Bus Selector3/2 -> Signal Conversion15/1  "<LM_OTLBufE2LastPNum>"
  Bus Selector3/1 -> Signal Conversion14/1  "<LM_OTLBufE2LastTPValid>"
  Bus Selector3/3 -> Signal Conversion16/1  "<LM_OTLBufE2LastSPPos>"
  Bus Selector3/4 -> Signal Conversion17/1  "<LM_OTLBufE2LastEPPos>"
  Signal Conversion14/1 -> LM_OTL_BufE2LastTPInfoAdju/3
  Signal Conversion15/1 -> LM_OTL_BufE2LastTPInfoAdju/4
  Signal Conversion16/1 -> LM_OTL_BufE2LastTPInfoAdju/5
  Signal Conversion17/1 -> LM_OTL_BufE2LastTPInfoAdju/6
  Signal Conversion23/1 -> LM_OTL_BufR1LastTPInfoAdju/6
  Signal Conversion22/1 -> LM_OTL_BufR1LastTPInfoAdju/5
  Signal Conversion21/1 -> LM_OTL_BufR1LastTPInfoAdju/4
  Signal Conversion20/1 -> LM_OTL_BufR1LastTPInfoAdju/3
  Bus Selector4/4 -> Signal Conversion23/1  "<LM_OTLBufR1LastEPPos>"
  Bus Selector4/3 -> Signal Conversion22/1  "<LM_OTLBufR1LastSPPos>"
  Bus Selector4/1 -> Signal Conversion20/1  "<LM_OTLBufR1LastTPValid>"
  Bus Selector4/2 -> Signal Conversion21/1  "<LM_OTLBufR1LastPNum>"
  Signal Conversion18/1 -> LM_OTL_BufR1LastTPInfoAdju/1
  Signal Conversion19/1 -> LM_OTL_BufR1LastTPInfoAdju/2
  Signal Conversion25/1 -> LM_OTL_BufR2LastTPInfoAdju/2
  Signal Conversion24/1 -> LM_OTL_BufR2LastTPInfoAdju/1
  LM_OTLBufLastTPInfoBus/1 -> Bus Selector/1, Bus Selector1/1, Bus Selector2/1, Bus Selector3/1, Bus Selector4/1, Bus Selector5/1
  Bus Selector5/2 -> Signal Conversion27/1  "<LM_OTLBufR2LastPNum>"
  Bus Selector5/1 -> Signal Conversion26/1  "<LM_OTLBufR2LastTPValid>"
  Bus Selector5/3 -> Signal Conversion28/1  "<LM_OTLBufR2LastSPPos>"
  Bus Selector5/4 -> Signal Conversion29/1  "<LM_OTLBufR2LastEPPos>"
  Signal Conversion26/1 -> LM_OTL_BufR2LastTPInfoAdju/3
  Signal Conversion27/1 -> LM_OTL_BufR2LastTPInfoAdju/4
  Signal Conversion28/1 -> LM_OTL_BufR2LastTPInfoAdju/5
  Signal Conversion29/1 -> LM_OTL_BufR2LastTPInfoAdju/6
  Signal Conversion30/1 -> LM_OTL_BufL1LastTPInfoAdju/1
  Signal Conversion31/1 -> LM_OTL_BufL1LastTPInfoAdju/2
  Signal Conversion32/1 -> LM_OTL_BufL1LastTPInfoAdju/3
  Signal Conversion33/1 -> LM_OTL_BufL1LastTPInfoAdju/4
  Signal Conversion34/1 -> LM_OTL_BufL1LastTPInfoAdju/5
  Signal Conversion35/1 -> LM_OTL_BufL1LastTPInfoAdju/6
  LM_OTL_BufL1LastTPInfoAdju/1 -> Signal Conversion36/1
  LM_OTL_BufL1LastTPInfoAdju/2 -> Signal Conversion37/1
  LM_OTL_BufL1LastTPInfoAdju/3 -> Signal Conversion38/1
  LM_OTL_BufL1LastTPInfoAdju/4 -> Signal Conversion39/1
  LM_OTL_BufL2LastTPInfoAdju/1 -> Signal Conversion40/1
  LM_OTL_BufL2LastTPInfoAdju/2 -> Signal Conversion41/1
  LM_OTL_BufL2LastTPInfoAdju/3 -> Signal Conversion42/1
  LM_OTL_BufL2LastTPInfoAdju/4 -> Signal Conversion43/1
  Signal Conversion36/1 -> Subsystem/1(LM_OTLBufL1LastTPValidAdju)
  Signal Conversion37/1 -> Subsystem/2(LM_OTLBufL1LastPNumAdju)
  Signal Conversion38/1 -> Subsystem/3(LM_OTLBufL1LastSPPosAdju)
  Signal Conversion39/1 -> Subsystem/4(LM_OTLBufL1LastEPPosAdju)
  Signal Conversion40/1 -> Subsystem/5(LM_OTLBufL2LastTPValidAdju)
  Signal Conversion41/1 -> Subsystem/6(LM_OTLBufL2LastPNumAdju)
  Signal Conversion42/1 -> Subsystem/7(LM_OTLBufL2LastSPPosAdju)
  Signal Conversion43/1 -> Subsystem/8(LM_OTLBufL2LastEPPosAdju)
  LM_OTL_BufE1LastTPInfoAdju/1 -> Signal Conversion44/1
  LM_OTL_BufE1LastTPInfoAdju/2 -> Signal Conversion45/1
  LM_OTL_BufE1LastTPInfoAdju/3 -> Signal Conversion46/1
  LM_OTL_BufE1LastTPInfoAdju/4 -> Signal Conversion47/1
  LM_OTL_BufE2LastTPInfoAdju/1 -> Signal Conversion48/1
  LM_OTL_BufE2LastTPInfoAdju/2 -> Signal Conversion49/1
  LM_OTL_BufE2LastTPInfoAdju/3 -> Signal Conversion50/1
  LM_OTL_BufE2LastTPInfoAdju/4 -> Signal Conversion51/1
  LM_OTL_BufR1LastTPInfoAdju/1 -> Signal Conversion52/1
  LM_OTL_BufR1LastTPInfoAdju/2 -> Signal Conversion53/1
  LM_OTL_BufR1LastTPInfoAdju/3 -> Signal Conversion54/1
  LM_OTL_BufR1LastTPInfoAdju/4 -> Signal Conversion55/1
  LM_OTL_BufR2LastTPInfoAdju/1 -> Signal Conversion56/1
  LM_OTL_BufR2LastTPInfoAdju/2 -> Signal Conversion57/1
  LM_OTL_BufR2LastTPInfoAdju/3 -> Signal Conversion58/1
  LM_OTL_BufR2LastTPInfoAdju/4 -> Signal Conversion59/1
  Signal Conversion44/1 -> Subsystem/9(LM_OTLBufE1LastTPValidAdju)
  Signal Conversion46/1 -> Subsystem/11(LM_OTLBufE1LastSPPosAdju)
  Signal Conversion45/1 -> Subsystem/10(LM_OTLBufE1LastPNumAdju)
  Signal Conversion47/1 -> Subsystem/12(LM_OTLBufE1LastEPPosAdju)
  Signal Conversion48/1 -> Subsystem/13(LM_OTLBufE2LastTPValidAdju)
  Signal Conversion49/1 -> Subsystem/14(LM_OTLBufE2LastPNumAdju)
  Signal Conversion51/1 -> Subsystem/16(LM_OTLBufE2LastEPPosAdju)
  Signal Conversion50/1 -> Subsystem/15(LM_OTLBufE2LastSPPosAdju)
  Signal Conversion52/1 -> Subsystem/17(LM_OTLBufR1LastTPValidAdju)
  Signal Conversion53/1 -> Subsystem/18(LM_OTLBufR1LastPNumAdju)
  Signal Conversion54/1 -> Subsystem/19(LM_OTLBufR1LastSPPosAdju)
  Signal Conversion55/1 -> Subsystem/20(LM_OTLBufR1LastEPPosAdju)
  Signal Conversion57/1 -> Subsystem/22(LM_OTLBufR2LastPNumAdju)
  Signal Conversion56/1 -> Subsystem/21(LM_OTLBufR2LastTPValidAdju)
  Signal Conversion58/1 -> Subsystem/23(LM_OTLBufR2LastSPPosAdju)
  Signal Conversion59/1 -> Subsystem/24(LM_OTLBufR2LastEPPosAdju)
  Subsystem/3(LM_OTLBufLastSPPosInfo) -> LM_OTLBufLastSPPosInfo/1
  Subsystem/2(LM_OTLBufLastPNumInfo) -> LM_OTLBufLastPNumInfo/1
  Subsystem/4(LM_OTLBufLastEPPosInfo) -> LM_OTLBufLastEPPosInfo/1
  Subsystem/1(LM_OTLBufLastTPValid) -> LM_OTLBufLastTPValid/1

== system PubIfDecisionLM_MDL/Subsystem2/LM_OTL/LM_OTL_MovObjTrajRecord3/LM_OTL_ObjStoreInfoCalc/Subsystem/LM_OTL_BufObjIDInfo ==
  LM_OTLBufL1ObjID : Inport
  LM_OTLBufL2ObjID : Inport  Port=2
  LM_OTLBufE1ObjID : Inport  Port=3
  LM_OTLBufE2ObjID : Inport  Port=4
  LM_OTLBufR1ObjID : Inport  Port=5
  LM_OTLBufR2ObjID : Inport  Port=6
  Bus Creator1 : BusCreator  Inputs=6
  LM_OTLBufObjIDInfo : Outport
  wires:
  LM_OTLBufR2ObjID/1 -> Bus Creator1/6  "LM_OTLBufR2ObjID"
  LM_OTLBufR1ObjID/1 -> Bus Creator1/5  "LM_OTLBufR1ObjID"
  LM_OTLBufE2ObjID/1 -> Bus Creator1/4  "LM_OTLBufE2ObjID"
  LM_OTLBufE1ObjID/1 -> Bus Creator1/3  "LM_OTLBufE1ObjID"
  LM_OTLBufL2ObjID/1 -> Bus Creator1/2  "LM_OTLBufL2ObjID"
  LM_OTLBufL1ObjID/1 -> Bus Creator1/1  "LM_OTLBufL1ObjID"
  Bus Creator1/1 -> LM_OTLBufObjIDInfo/1  "LM_OTLBufObjIDInfo"

== system PubIfDecisionLM_MDL/Subsystem2/LM_OTL/LM_OTL_MovObjTrajRecord3/LM_OTL_ObjStoreInfoCalc/Subsystem/LM_OTL_BufPNumInfo ==
  LM_OTLBufL1ObjTPNum : Inport
  LM_OTLBufL2ObjTPNum : Inport  Port=2
  LM_OTLBufE1ObjTPNum : Inport  Port=3
  LM_OTLBufE2ObjTPNum : Inport  Port=4
  LM_OTLBufR1ObjTPNum : Inport  Port=5
  LM_OTLBufR2ObjTPNum : Inport  Port=6
  Bus Creator2 : BusCreator  Inputs=6
  LM_OTLBufPNumInfo : Outport
  wires:
  Bus Creator2/1 -> LM_OTLBufPNumInfo/1  "LM_OTLBufPNumInfo"
  LM_OTLBufL1ObjTPNum/1 -> Bus Creator2/1  "LM_OTLBufL1PNum"
  LM_OTLBufR2ObjTPNum/1 -> Bus Creator2/6  "LM_OTLBufR2PNum"
  LM_OTLBufR1ObjTPNum/1 -> Bus Creator2/5  "LM_OTLBufR1PNum"
  LM_OTLBufL2ObjTPNum/1 -> Bus Creator2/2  "LM_OTLBufL2PNum"
  LM_OTLBufE2ObjTPNum/1 -> Bus Creator2/4  "LM_OTLBufE2PNum"
  LM_OTLBufE1ObjTPNum/1 -> Bus Creator2/3  "LM_OTLBufE1PNum"

== system PubIfDecisionLM_MDL/Subsystem2/LM_OTL/LM_OTL_MovObjTrajRecord3/LM_OTL_ObjStoreInfoCalc/Subsystem/LM_OTL_BufSPPosInfo ==
  LM_OTLBufL1SPPos : Inport
  LM_OTLBufL2SPPos : Inport  Port=2
  LM_OTLBufE1SPPos : Inport  Port=3
  LM_OTLBufLE2SPPos : Inport  Port=4
  LM_OTLBufR1SPPos : Inport  Port=5
  LM_OTLBufR2SPPos : Inport  Port=6
  Bus Creator3 : BusCreator  Inputs=6
  LM_OTLBufSPPosInfo : Outport
  wires:
  LM_OTLBufR1SPPos/1 -> Bus Creator3/5  "LM_OTLBufR1SPPos"
  LM_OTLBufL2SPPos/1 -> Bus Creator3/2  "LM_OTLBufL2SPPos"
  LM_OTLBufLE2SPPos/1 -> Bus Creator3/4  "LM_OTLBufE2SPPos"
  LM_OTLBufE1SPPos/1 -> Bus Creator3/3  "LM_OTLBufE1SPPos"
  Bus Creator3/1 -> LM_OTLBufSPPosInfo/1  "LM_OTLBufSPPosInfo"
  LM_OTLBufR2SPPos/1 -> Bus Creator3/6  "LM_OTLBufR2SPPos"
  LM_OTLBufL1SPPos/1 -> Bus Creator3/1  "LM_OTLBufL1SPPos"

== system PubIfDecisionLM_MDL/Subsystem2/LM_OTL/LM_OTL_MovObjTrajRecord3/LM_OTL_ObjStoreInfoCalc/Subsystem/LM_OTL_BufTPVectInfo ==
  LM_OTLBufL1DxVect : Inport
  LM_OTLBufL1DyVect : Inport  Port=2
  LM_OTLBufL2DxVect : Inport  Port=3
  LM_OTLBufL2DyVect : Inport  Port=4
  LM_OTLBufE1DxVect : Inport  Port=5
  LM_OTLBufE1DyVect : Inport  Port=6
  LM_OTLBufE2DxVect : Inport  Port=7
  LM_OTLBufE2DyVect : Inport  Port=8
  LM_OTLBufR1DxVect : Inport  Port=9
  LM_OTLBufR1DyVect : Inport  Port=10
  LM_OTLBufR2DxVect : Inport  Port=11
  LM_OTLBufR2DyVect : Inport  Port=12
  Bus Creator : BusCreator  Inputs=12
  LM_OTLBufTPVectBus : Outport
  wires:
  Bus Creator/1 -> LM_OTLBufTPVectBus/1  "LM_OTLBufTPVectBus"
  LM_OTLBufR2DyVect/1 -> Bus Creator/12  "LM_OTLBufR2DyVect"
  LM_OTLBufR2DxVect/1 -> Bus Creator/11  "LM_OTLBufR2DxVect"
  LM_OTLBufR1DyVect/1 -> Bus Creator/10  "LM_OTLBufR1DyVect"
  LM_OTLBufR1DxVect/1 -> Bus Creator/9  "LM_OTLBufR1DxVect"
  LM_OTLBufE2DyVect/1 -> Bus Creator/8  "LM_OTLBufE2DyVect"
  LM_OTLBufE2DxVect/1 -> Bus Creator/7  "LM_OTLBufE2DxVect"
  LM_OTLBufE1DyVect/1 -> Bus Creator/6  "LM_OTLBufE1DyVect"
  LM_OTLBufE1DxVect/1 -> Bus Creator/5  "LM_OTLBufE1DxVect"
  LM_OTLBufL2DyVect/1 -> Bus Creator/4  "LM_OTLBufL2DyVect"
  LM_OTLBufL2DxVect/1 -> Bus Creator/3  "LM_OTLBufL2DxVect"
  LM_OTLBufL1DyVect/1 -> Bus Creator/2  "LM_OTLBufL1DyVect"
  LM_OTLBufL1DxVect/1 -> Bus Creator/1  "LM_OTLBufL1DxVect"

== system PubIfDecisionLM_MDL/Subsystem2/LM_OTL/LM_OTL_MovObjTrajRecord3/LM_OTL_ObjStoreInfoCalc/Subsystem/Subsystem1 ==
  LM_OTLBufObjIDInfo : Inport
  LM_OTLBufPNumInfo : Inport  Port=2
  LM_OTLBufSPPosInfo : Inport  Port=3
  LM_OTLBufEPPosInfo : Inport  Port=4
  LM_OTLBufLastTPValid : Inport  Port=5
  LM_OTLBufLastPNumInfo : Inport  Port=6
  LM_OTLBufLastSPPosInfo : Inport  Port=7
  LM_OTLBufLastEPPosInfo : Inport  Port=8
  Bus Creator : BusCreator  Inputs=8
  LM_OTLBufTPInfoBus : Outport
  wires:
  LM_OTLBufObjIDInfo/1 -> Bus Creator/1
  LM_OTLBufPNumInfo/1 -> Bus Creator/2
  LM_OTLBufSPPosInfo/1 -> Bus Creator/3
  LM_OTLBufEPPosInfo/1 -> Bus Creator/4
  LM_OTLBufLastTPValid/1 -> Bus Creator/5
  LM_OTLBufLastPNumInfo/1 -> Bus Creator/6
  LM_OTLBufLastSPPosInfo/1 -> Bus Creator/7
  LM_OTLBufLastEPPosInfo/1 -> Bus Creator/8
  Bus Creator/1 -> LM_OTLBufTPInfoBus/1  "LM_OTLBufTPInfoBus"

== system PubIfDecisionLM_MDL/Subsystem2/LM_VSL/LM_VSLFntPath/LM_VSL_LineInfoEvalutaion/LM_VSL_BaseLinePCalc3/Subsystem ==
  LM_VSLLineMaxQualityIndex : Inport
  LM_VSLLineMinQualityIndex : Inport  Port=2
  LM_ComLineLostNum : Inport  Port=3
  LM_VSLLineC1Vect : Inport  Port=4
  LM_VSLLineC2Vect : Inport  Port=5
  LM_VSLLineC3Vect : Inport  Port=6
  LM_VSLLineQualityVect : Inport  Port=7
  Diffnum : Inport  Port=8
  LM_VSLDiffValid : Inport  Port=9
  LM_VSLMinQualityLineValid : Inport  Port=10
  LM_VSLLineDisFntVect : Inport  Port=11
  LM_VSLBLFntDis : Inport  Port=12
  Merge{,1..3} (4 alike) : Merge  Inputs=4
  Switch Case : SwitchCase  CaseConditions={[0,1],2,3,4}  ShowDefaultCase=off
  Switch Case Action Subsystem : Subsystem  TreatAsAtomicUnit=on
  Switch Case Action Subsystem1 : Subsystem  TreatAsAtomicUnit=on
  Switch Case Action Subsystem2 : Subsystem  TreatAsAtomicUnit=on
  Switch Case Action Subsystem3 : Subsystem  TreatAsAtomicUnit=on
  LM_VSLBaseC1 : Outport
  LM_VSLBaseC2 : Outport  Port=2
  LM_VSLBaseC3 : Outport  Port=3
  LM_VSLBaseQuality : Outport  Port=4
  wires:
  LM_VSLBLFntDis/1 -> Switch Case Action Subsystem/8(LM_VSLBLFntDis)
  LM_VSLLineDisFntVect/1 -> Switch Case Action Subsystem/7(LM_VSLLineDisFntVect)
  Merge2/1 -> LM_VSLBaseC3/1
  Merge1/1 -> LM_VSLBaseC2/1
  Merge/1 -> LM_VSLBaseC1/1
  Switch Case Action Subsystem1/3(LM_VSLBaseC3) -> Merge2/4
  Switch Case Action Subsystem2/3(LM_VSLBaseC3) -> Merge2/3
  Switch Case Action Subsystem1/1(LM_VSLBaseC1) -> Merge/4
  Switch Case Action Subsystem1/2(LM_VSLBaseC2) -> Merge1/4
  Switch Case Action Subsystem2/2(LM_VSLBaseC2) -> Merge1/3
  Switch Case Action Subsystem2/1(LM_VSLBaseC1) -> Merge/3
  Switch Case Action Subsystem/3(LM_VSLBaseC3) -> Merge2/2
  Switch Case Action Subsystem/2(LM_VSLBaseC2) -> Merge1/2
  Switch Case Action Subsystem/1(LM_VSLBaseC1) -> Merge/2
  Switch Case/4 -> Switch Case Action Subsystem1/Action
  LM_VSLLineMaxQualityIndex/1 -> Switch Case Action Subsystem2/5(LM_VSLLineMaxQualityIndex)
  LM_VSLMinQualityLineValid/1 -> Switch Case Action Subsystem/6(LM_VSLMinQualityLineValid), Switch Case Action Subsystem3/8(LM_VSLMinQualityLineValid)
  LM_VSLLineC1Vect/1 -> Switch Case Action Subsystem/2(LM_VSLLineC1Vect), Switch Case Action Subsystem2/1(LM_VSLLineC1Vect), Switch Case Action Subsystem3/4(LM_VSLLineC1Vect)
  LM_VSLLineMinQualityIndex/1 -> Switch Case Action Subsystem/1(LM_VSLLineMinQualityIndex), Switch Case Action Subsystem3/3(LM_VSLLineMinQualityIndex)
  LM_VSLLineQualityVect/1 -> Switch Case Action Subsystem/5(LM_VSLLineQualityVect), Switch Case Action Subsystem2/4(LM_VSLLineQualityVect), Switch Case Action Subsystem3/7(LM_VSLLineQualityVect)
  LM_VSLLineC2Vect/1 -> Switch Case Action Subsystem/3(LM_VSLLineC2Vect), Switch Case Action Subsystem2/2(LM_VSLLineC2Vect), Switch Case Action Subsystem3/5(LM_VSLLineC2Vect)
  LM_VSLLineC3Vect/1 -> Switch Case Action Subsystem/4(LM_VSLLineC3Vect), Switch Case Action Subsystem2/3(LM_VSLLineC3Vect), Switch Case Action Subsystem3/6(LM_VSLLineC3Vect)
  Switch Case/3 -> Switch Case Action Subsystem2/Action
  Switch Case/2 -> Switch Case Action Subsystem/Action
  LM_ComLineLostNum/1 -> Switch Case/1
  Switch Case/1 -> Switch Case Action Subsystem3/Action
  LM_VSLDiffValid/1 -> Switch Case Action Subsystem3/2(LM_VSLDiffValid)
  Diffnum/1 -> Switch Case Action Subsystem3/1(Diffnum)
  Switch Case Action Subsystem3/1(LM_VSLBaseC1) -> Merge/1
  Switch Case Action Subsystem3/2(LM_VSLBaseC2) -> Merge1/1
  Switch Case Action Subsystem3/3(LM_VSLBaseC3) -> Merge2/1
  Switch Case Action Subsystem3/4(LM_VSLBaseQuality) -> Merge3/1
  Switch Case Action Subsystem/4(LM_VSLBaseQuality) -> Merge3/2
  Switch Case Action Subsystem2/4(LM_VSLBaseQuality) -> Merge3/3
  Switch Case Action Subsystem1/4(LM_VSLBaseQuality) -> Merge3/4
  Merge3/1 -> LM_VSLBaseQuality/1
